simulink model "myFOC"  (R2024b)
settings: Solver=VariableStepAuto  StartTime=0.0  StopTime=6  RelTol=1e-3
InitFcn:
  | init_param;
undefined symbols (not defined in the file): DiscIntNeverNeededParam, inverter, Ki_id, Ki_iq, Kp_id, Kp_iq, PI_params, pmsm, Ts, Ts_motor, Ts_simulink
libraries: mcbcontrolslib x8, simulink x3, slpidlib x1, mcbpmsmnonlinearlib x1, autolibpmsminterior x1
settings Model: Creator=RUSHI JARIWALA  LastModifiedBy=admin
settings SolverCC: AlgebraicLoopSolver=TrustRegion
settings DebuggingCC: UnconnectedInputMsg=warning  UnconnectedOutputMsg=warning  UnconnectedLineMsg=warning
settings ModelReferenceCC: EnableRefExpFcnMdlSchedulingChecks=on
settings RTWCC: GPUComputeCapability=3.5

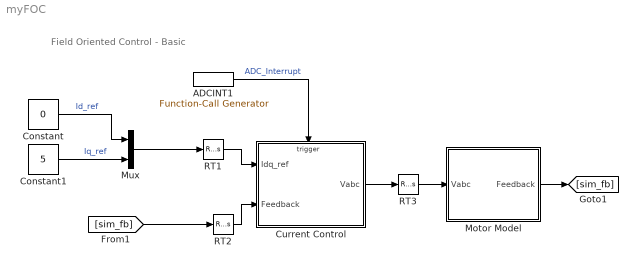
== system myFOC ==
  note: Field Oriented Control - Basic
  ADCINT1 : simulink/Ports & Subsystems/Function-Call Generator  sample_time=Ts  numberOfIterations=1  DisallowWideOutput=off
  Constant : Constant  Value=0  OutDataTypeStr=single
  Constant1 : Constant  Value=5  OutDataTypeStr=single
  Current Control : Subsystem
      settings: RTWSystemCode=Nonreusable function
  Motor Model : Subsystem
  Mux : Mux  Inputs=2
  RT1 : RateTransition  Deterministic=off
  RT2 : RateTransition  Deterministic=off
  RT3 : RateTransition  Deterministic=off
  wires:
  RT2/1 -> Current Control/2(Feedback)
  RT1/1 -> Current Control/1(Idq_ref)
  [sim_fb] -> RT2/1
  Mux/1 -> RT1/1
  Constant/1 -> Mux/1  "Id_ref"
  RT3/1 -> Motor Model/1(Vabc)
  Motor Model/1(Feedback) -> [sim_fb]
  Current Control/1(Vabc) -> RT3/1
  Constant1/1 -> Mux/2  "Iq_ref"
  ADCINT1/1 -> Current Control/Trigger  "ADC_Interrupt"

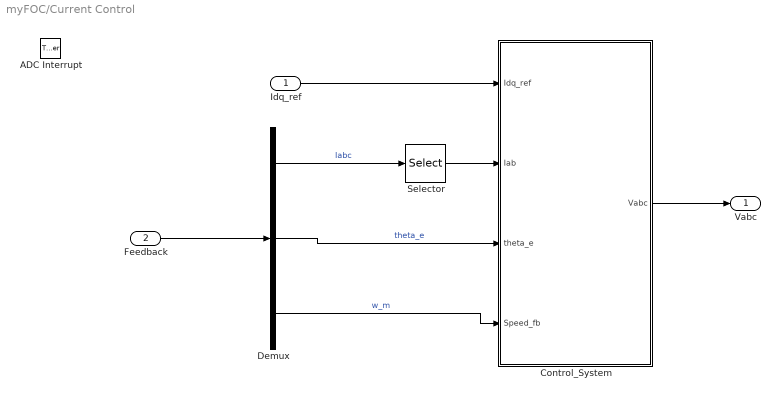
== system myFOC/Current Control ==
  Idq_ref : Inport
  Feedback : Inport  Port=2
  ADC Interrupt : TriggerPort  TriggerType=function-call  VariantControl=Variant
  Control_System : Subsystem
  Demux : Demux  Outputs=3
      settings: DisplayOption=none
  Selector : Selector  InputPortWidth=3  IndexOptions=Index vector (dialog)  Indices=[1 2]  OutputSizes=1
  Vabc : Outport  InitialOutput=0  VectorParamsAs1DForOutWhenUnconnected=off
  wires:
  Idq_ref/1 -> Control_System/1(Idq_ref)
  Control_System/1(Vabc) -> Vabc/1
  Demux/3 -> Control_System/4(Speed_fb)  "w_m"
  Feedback/1 -> Demux/1
  Demux/2 -> Control_System/3(theta_e)  "theta_e"
  Demux/1 -> Selector/1  "Iabc"
  Selector/1 -> Control_System/2(Iab)

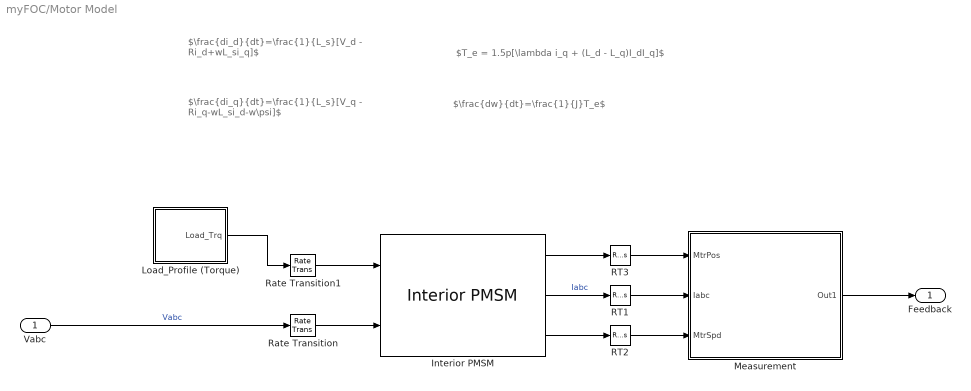
== system myFOC/Motor Model ==
  note: $\frac{dw}{dt}=\frac{1}{J}T_e$
  note: $\frac{di_d}{dt}=\frac{1}{L_s}[V_d - Ri_d+wL_si_q]$
  note: $\frac{di_q}{dt}=\frac{1}{L_s}[V_q - Ri_q-wL_si_d-w\psi]$
  note: $T_e = 1.5p[\lambda i_q + (L_d - L_q)I_dI_q]$
  Vabc : Inport
  Interior PMSM : autolibpmsminterior/Interior PMSM  port_config=Torque  sim_type=Discrete  Ts=Ts_motor  P=pmsm.p  Rs=pmsm.Rs  Ldq=[pmsm.Ld pmsm.Lq]  KConstText=Permanent flux linkage constant (lambda_pm):  lambda_pm=pmsm.FluxPM  Ke=159.9771  mechanical=[pmsm.J, pmsm.B,0]  idq0=[0 0]  theta_init=0  omega_init=0  KConst=pmsm.FluxPM  lambda_pm_calc=pmsm.FluxPM  Kt=0.07  RefBlkName='autolibpmsminterior/Interior PMSM'  aMode=5
      settings: LibrarySourceBlock=mcblib/Electrical Systems/Motors/Interior PMSM
  Load_Profile (Torque) : Subsystem
  Measurement : Subsystem
  RT1 : RateTransition  Deterministic=off  OutPortSampleTime=Ts_simulink
  RT2 : RateTransition  Deterministic=off  OutPortSampleTime=Ts_simulink
  RT3 : RateTransition  Deterministic=off  OutPortSampleTime=Ts_simulink
  Rate Transition : RateTransition  Deterministic=off  OutPortSampleTime=Ts_motor
  Rate Transition1 : RateTransition  Deterministic=off  OutPortSampleTime=Ts_motor
  Feedback : Outport  VectorParamsAs1DForOutWhenUnconnected=off
  wires:
  Measurement/1(Out1) -> Feedback/1
  Interior PMSM/3 -> RT2/1
  RT2/1 -> Measurement/3(MtrSpd)
  RT1/1 -> Measurement/2(Iabc)
  RT3/1 -> Measurement/1(MtrPos)
  Interior PMSM/1 -> RT3/1
  Rate Transition/1 -> Interior PMSM/2
  Vabc/1 -> Rate Transition/1  "Vabc"
  Interior PMSM/2 -> RT1/1  "Iabc"
  Rate Transition1/1 -> Interior PMSM/1
  Load_Profile (Torque)/1(Load_Trq) -> Rate Transition1/1

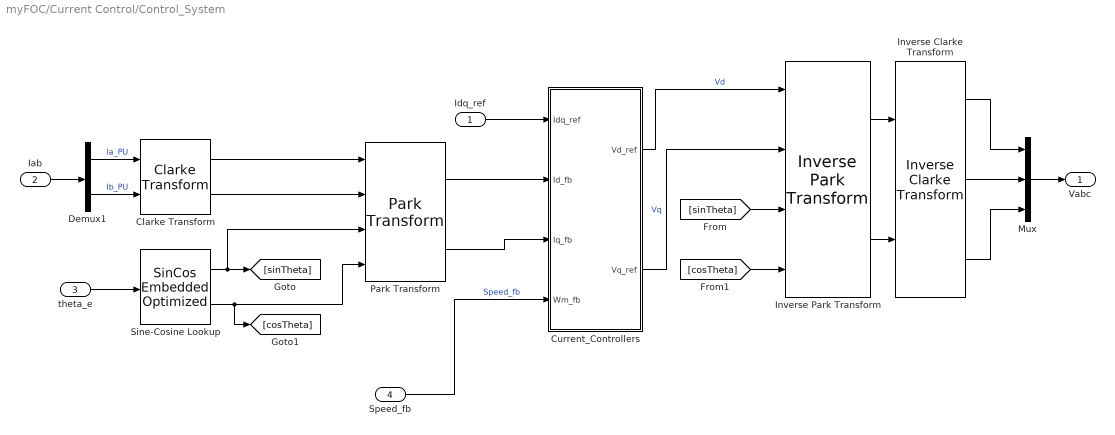
== system myFOC/Current Control/Control_System ==
  Idq_ref : Inport
  Iab : Inport  Port=2
  theta_e : Inport  Port=3
  Speed_fb : Inport  Port=4
  Clarke Transform : mcbcontrolslib/Clarke Transform  VariantControl=Variant2  PhaseInput=Two inputs  EnPowerInv=off
  Current_Controllers : Subsystem
  Demux1 : Demux  Outputs=2
  Inverse Clarke Transform : mcbcontrolslib/Inverse Clarke Transform  PhaseInput=Two inputs  EnPowerInv=off
  Inverse Park Transform : mcbcontrolslib/Inverse Park Transform  PhaseInput=Two inputs  AxisAlignment=D-axis  ThetaInput=Sine and Cosine electrical position  AngleInput=Per-unit  N_points=1024
  Mux : Mux  Inputs=3
  Park Transform : mcbcontrolslib/Park Transform  PhaseInput=Two inputs  AxisAlignment=D-axis  ThetaInput=Sine and Cosine electrical position  AngleInput=Per-unit  N_points=1024
  Sine-Cosine Lookup : mcbcontrolslib/SinCos Embedded Optimized  LabelModeActiveChoice=MCB_Sin  OptforProc=off  ApproximationMethod=None  UserApproxMethod=Lookup  ApproxStatus=None  InterpMethod=Linear point-slope  NumberOfDataPoints=16  NumberOfIterations=11  RemoveProtectionAgainstOutOfRangeInput=off  TableDataTypeStr=Inherit: Inherit via input  AngleInput=Per-unit  ThetaDataType=single  N_points=1024  DatatypeInput=Inherit from input  Datatype=Inherit: Same as input
  Vabc : Outport
  wires:
  Park Transform/1 -> Current_Controllers/2(Id_fb)
  Park Transform/2 -> Current_Controllers/3(Iq_fb)
  Sine-Cosine Lookup/1 -> [sinTheta], Park Transform/3
  Sine-Cosine Lookup/2 -> Park Transform/4, [cosTheta]
  [cosTheta] -> Inverse Park Transform/4
  [sinTheta] -> Inverse Park Transform/3
  Clarke Transform/2 -> Park Transform/2
  Clarke Transform/1 -> Park Transform/1
  Idq_ref/1 -> Current_Controllers/1(Idq_ref)
  Current_Controllers/1(Vd_ref) -> Inverse Park Transform/1  "Vd"
  Current_Controllers/2(Vq_ref) -> Inverse Park Transform/2  "Vq"
  Demux1/1 -> Clarke Transform/1  "Ia_PU"
  Demux1/2 -> Clarke Transform/2  "Ib_PU"
  Iab/1 -> Demux1/1
  Speed_fb/1 -> Current_Controllers/4(Wm_fb)  "Speed_fb"
  theta_e/1 -> Sine-Cosine Lookup/1
  Inverse Park Transform/1 -> Inverse Clarke Transform/1
  Inverse Park Transform/2 -> Inverse Clarke Transform/2
  Inverse Clarke Transform/1 -> Mux/1
  Inverse Clarke Transform/2 -> Mux/2
  Inverse Clarke Transform/3 -> Mux/3
  Mux/1 -> Vabc/1

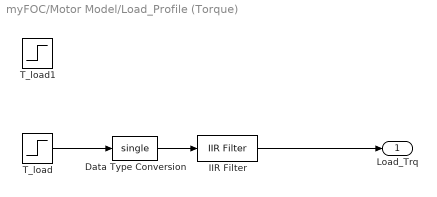
== system myFOC/Motor Model/Load_Profile (Torque) ==
  Data Type Conversion : DataTypeConversion  OutDataTypeStr=single  SaturateOnIntegerOverflow=off  RndMeth=Floor
  IIR Filter : mcbcontrolslib/IIR Filter  VariantControl=Low Pass Filter  VariantSelect=Low-pass  FilterConstantInputType=Specify via dialog  Filter_constant=0.01  advancedSettings=off  Ts=50e-6  cutOff_freq=32.1525
  T_load : Step  Time=5.5  Before=0*pmsm.T_rated  After=0*pmsm.T_rated  SampleTime=Ts_simulink
  T_load1 : Step  Time=2  Before=0.05*pmsm.T_rated  After=-0.05*pmsm.T_rated  SampleTime=Ts_simulink
  Load_Trq : Outport  VectorParamsAs1DForOutWhenUnconnected=off
  wires:
  T_load/1 -> Data Type Conversion/1
  Data Type Conversion/1 -> IIR Filter/1
  IIR Filter/1 -> Load_Trq/1

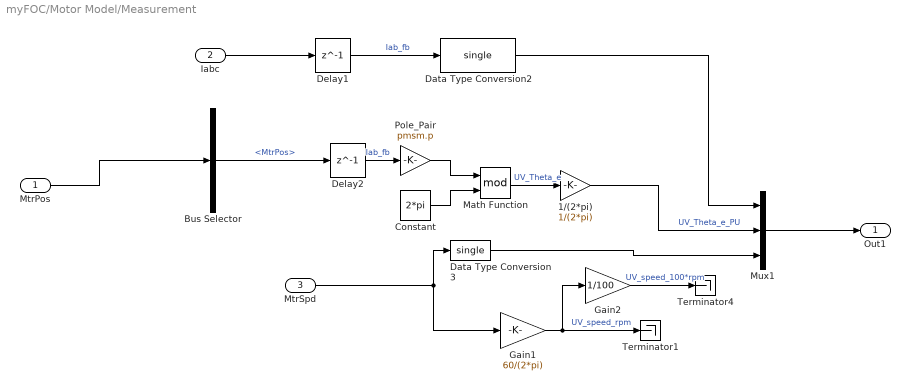
== system myFOC/Motor Model/Measurement ==
  MtrPos : Inport
  Iabc : Inport  Port=2
  MtrSpd : Inport  Port=3
  1/(2*pi) : Gain  Gain=1/(2*pi)  OutDataTypeStr=dataType
  Bus Selector : BusSelector  OutputSignals=MtrPos
  Constant : Constant  Value=2*pi  SampleTime=-1
  Data Type Conversion2 : DataTypeConversion  OutDataTypeStr=single  SaturateOnIntegerOverflow=off  RndMeth=Floor
  Data Type Conversion3 : DataTypeConversion  OutDataTypeStr=single  SaturateOnIntegerOverflow=off  RndMeth=Floor
  Delay1 : Delay  DelayLength=1
  Delay2 : Delay  DelayLength=1
  Gain1 : Gain  Gain=60/(2*pi)  OutDataTypeStr=dataType
  Gain2 : Gain  Gain=1/100  OutDataTypeStr=dataType
  Math Function : Math  Operator=mod
  Mux1 : Mux  Inputs=3
  Pole_Pair : Gain  Gain=pmsm.p
  Terminator1 : Terminator
  Terminator4 : Terminator
  Out1 : Outport
  wires:
  Delay1/1 -> Data Type Conversion2/1  "Iab_fb"
  Delay2/1 -> Pole_Pair/1  "Iab_fb"
  Bus Selector/1 -> Delay2/1  "<MtrPos>"
  Pole_Pair/1 -> Math Function/1
  Constant/1 -> Math Function/2
  Math Function/1 -> 1/(2*pi)/1  "UV_Theta_e"
  1/(2*pi)/1 -> Mux1/2  "UV_Theta_e_PU"
  Mux1/1 -> Out1/1
  MtrSpd/1 -> Gain1/1, Data Type Conversion3/1
  Iabc/1 -> Delay1/1
  MtrPos/1 -> Bus Selector/1
  Gain1/1 -> Gain2/1, Terminator1/1  "UV_speed_rpm"
  Data Type Conversion3/1 -> Mux1/3
  Data Type Conversion2/1 -> Mux1/1
  Gain2/1 -> Terminator4/1  "UV_speed_100*rpm"

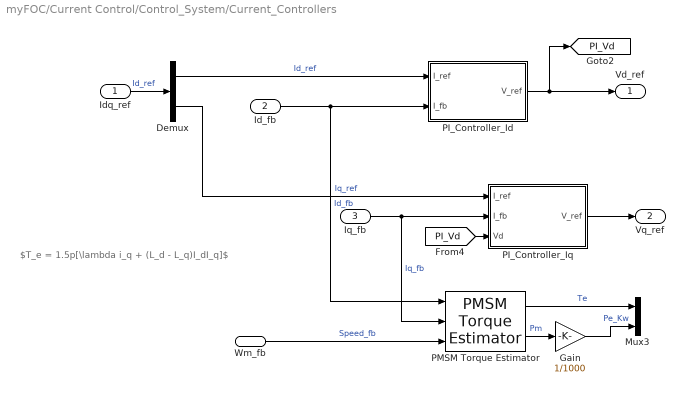
== system myFOC/Current Control/Control_System/Current_Controllers ==
  note: $T_e = 1.5p[\lambda i_q + (L_d - L_q)I_dI_q]$
  Idq_ref : Inport
  Id_fb : Inport  Port=2
  Iq_fb : Inport  Port=3
  Wm_fb : Inport  Port=4
  Demux : Demux  Outputs=2
  Gain : Gain  Gain=1/1000
  Mux3 : Mux  Inputs=2
  PI_Controller_Id : Subsystem
  PI_Controller_Iq : Subsystem
  PMSM Torque Estimator : mcbpmsmnonlinearlib/PMSM Torque Estimator  polePairs=pmsm.p  nonLinearityChoice=Linear model with lumped parameters  Ld=pmsm.Ld  Lq=pmsm.Lq  FluxPM=pmsm.FluxPM  idVec=[-40, -20, 0, 20]  iqVec=[-40, -20, 0, 20, 40]  LdTable=0.2e-3 * ones(4, 5)  LqTable=0.2e-3 * ones(4, 5)  FluxPMTable=6.4e-3 * ones(4, 5)  FluxDTable=[-1.6,-1.6,-1.6,-1.6,-1.6;2.4,2.4,2.4,2.4,2.4;6.4,6.4,6.4,6.4,6.4;10.4,10.4,10.4,10.4,10.4]*1e-3  FluxQTable=[-8,-4,0,4,8;-8,-4,0,4,8;-8,-4,0,4,8;-8,-4,0,4,8]*1e-3  Units=SI Units  V_base=PU_System.V_base  I_base=PU_System.I_base  N_base=PU_System.N_base  T_base=1  P_base=1  scaledTables=on
  Vd_ref : Outport  VectorParamsAs1DForOutWhenUnconnected=off
  Vq_ref : Outport  Port=2  VectorParamsAs1DForOutWhenUnconnected=off
  tag scope: PI_Vd=global
  wires:
  Id_fb/1 -> PMSM Torque Estimator/1, PI_Controller_Id/2(I_fb)  "Id_fb"
  PI_Controller_Iq/1(V_ref) -> Vq_ref/1
  PMSM Torque Estimator/1 -> Mux3/1  "Te"
  Iq_fb/1 -> PMSM Torque Estimator/2, PI_Controller_Iq/2(I_fb)  "Iq_fb"
  Idq_ref/1 -> Demux/1  "Id_ref"
  Wm_fb/1 -> PMSM Torque Estimator/3  "Speed_fb"
  Demux/1 -> PI_Controller_Id/1(I_ref)  "Id_ref"
  Demux/2 -> PI_Controller_Iq/1(I_ref)  "Iq_ref"
  [PI_Vd] -> PI_Controller_Iq/3(Vd)
  PMSM Torque Estimator/2 -> Gain/1  "Pm"
  Gain/1 -> Mux3/2  "Pe_Kw"
  PI_Controller_Id/1(V_ref) -> Vd_ref/1, [PI_Vd]

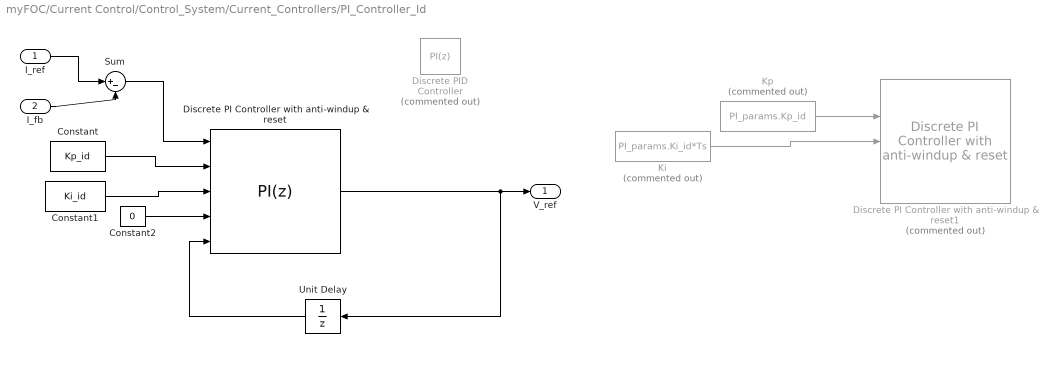
== system myFOC/Current Control/Control_System/Current_Controllers/PI_Controller_Id ==
  I_ref : Inport
  I_fb : Inport  Port=2
  Constant : Constant  Value=Kp_id  OutDataTypeStr=single  SampleTime=-1
  Constant1 : Constant  Value=Ki_id  OutDataTypeStr=single  SampleTime=-1
  Constant2 : Constant  Value=0
  Discrete PI Controller with anti-windup & reset : slpidlib/PID Controller  Controller=PI  Form=Parallel  TimeDomain=Discrete-time  UseExternalTs=off  SampleTime=-1  IntegratorMethod=Forward Euler  FilterMethod=Forward Euler  ControllerParametersSource=external  P=1  I=1  UseKiTs=on  D=0  UseExternalDerivativeSource=off  N=100  UseFilter=on  TunerSelectOption=Transfer Function Based (PID Tuner App)  InitialConditionSource=external  InitialConditionForIntegrator=0  InitialConditionForFilter=0  DifferentiatorICPrevScaledInput=0  ExternalReset=level  TrackingMode=off  Kt=1  LimitOutput=on  SatLimitsSource=internal  UpperSaturationLimit=0.95*inverter.V_dc/sqrt(3)  LowerSaturationLimit=-0.95*inverter.V_dc/sqrt(3)  LinearizeAsGain=on  AntiWindupMode=clamping  Kb=1  LimitIntegrator=off  UpperIntegratorSaturationLimit=inf  LowerIntegratorSaturationLimit=-inf  RndMeth=Simplest  POutMin=[]  POutMax=[]  IOutMin=[]  IOutMax=[]  DOutMin=[]  DOutMax=[]  NOutMin=[]  NOutMax=[]  SumOutMin=[]  SumOutMax=[]  SaturationOutDataTypeStr=Inherit: Inherit via back propagation  SaturationOutMin=[]  SaturationOutMax=[]  PParamMin=[]  PParamMax=[]  IParamMin=[]  IParamMax=[]  DParamMin=[]  DParamMax=[]  NParamMin=[]  NParamMax=[]  KbParamMin=[]  KbParamMax=[]  KtParamMin=[]  KtParamMax=[]  KbOutMin=[]  KbOutMax=[]  KtOutMin=[]  KtOutMax=[]  IntegratorOutMin=[]  IntegratorOutMax=[]  FilterOutMin=[]  FilterOutMax=[]  SumI1OutMin=[]  SumI1OutMax=[]  SumI2OutMin=[]  SumI2OutMax=[]  SumI3OutMin=[]  SumI3OutMax=[]  SumI4OutMin=[]  SumI4OutMax=[]  SumDOutMin=[]  SumDOutMax=[]  DifferentiatorOutMin=[]  DifferentiatorOutMax=[]  FilterDiffOutCoefMin=[]  FilterDiffOutCoefMax=[]  ReciprocalOutMin=[]  ReciprocalOutMax=[]  SumDenOutMin=[]  SumDenOutMax=[]  SumNumOutMin=[]  SumNumOutMax=[]  DivideOutMin=[]  DivideOutMax=[]  UdiffTsProdOutMin=[]  UdiffTsProdOutMax=[]  NTsProdOutMin=[]  NTsProdOutMax=[]  UintegralTsProdOutMin=[]  UintegralTsProdOutMax=[]  UngainTsProdOutMin=[]  UngainTsProdOutMax=[]  ClampingZeroOutDataTypeStr=Inherit: Inherit via back propagation  ClampingZeroOutMin=[]  ClampingZeroOutMax=[]  FilterDenConstantOutDataTypeStr=Inherit: Inherit via back propagation  FilterDenConstantOutMin=[]  FilterDenConstantOutMax=[]  PCopyOutDataTypeStr=Inherit: Inherit via back propagation  PCopyOutMin=[]  PCopyOutMax=[]  NCopyOutDataTypeStr=Inherit: Inherit via back propagation  NCopyOutMin=[]  NCopyOutMax=[]  IntegratorContinuousStateAttributes=''  IntegratorStateMustResolveToSignalObject=off  IntegratorRTWStateStorageClass=Auto  FilterContinuousStateAttributes=''  FilterStateMustResolveToSignalObject=off  FilterRTWStateStorageClass=Auto  ParallelPVariant=ExternalParameters  IdealPVariant=Disabled  IVariant=ExternalParameters  DVariant=Disabled  IntegratorVariant=Discrete  SatVariant=Enabled  AWVariant=DiscClampingParallel  PCopyVariant=Disabled  TRVariant=Disabled  FdbkBlocksVariant=Forward  IdealPFdbkVariant=Disabled  SatFdbkVariant=Disabled  DerivativeFilterVariant=Disabled  NVariant=Disabled  NCopyVariant=Disabled_SignalSpec  FilterICVariant=Disabled  IntegratorICVariant=ExternalICs  ExternalResetVariant=ExternalReset  TRSumVariant=Passthrough  SumFdbkVariant=Disabled  SumVariant=Sum_PI  TsampFilterVariant=InternalTs  TsampNgainVariant=Passthrough  TsampIntegralVariant=Disabled_SignalSpec  ExternalSaturationOutDataTypeStr=Inherit: Same as second input  DerivativeSourceVariant=Disabled  PreIntVariant=InternalPreInt
      settings: LibrarySourceBlock=mcbcontrolslib/PI Controller
  Discrete PI Controller with anti-windup & reset1 : mcbcontrolslib/Discrete PI Controller  with anti-windup & reset  Commented=on  UpperSaturationLimit=1  LowerSaturationLimit=-1
  Discrete PID Controller : simulink/Continuous/PID Controller  Commented=on  Controller=PI  Form=Parallel  TimeDomain=Discrete-time  UseExternalTs=off  SampleTime=-1  IntegratorMethod=Forward Euler  FilterMethod=Forward Euler  ControllerParametersSource=internal  P=1  I=1  D=0  UseFilter=on  N=100  TunerSelectOption=Transfer Function Based (PID Tuner App)  InitialConditionSource=internal  InitialConditionForIntegrator=0  InitialConditionForFilter=0  DifferentiatorICPrevScaledInput=0  ExternalReset=none  TrackingMode=off  Kt=1  LimitOutput=off  UpperSaturationLimit=inf  LowerSaturationLimit=-inf  LinearizeAsGain=off  AntiWindupMode=none  Kb=1  POutMin=[]  POutMax=[]  IOutMin=[]  IOutMax=[]  DOutMin=[]  DOutMax=[]  NOutMin=[]  NOutMax=[]  SumOutMin=[]  SumOutMax=[]  SaturationOutMin=[]  SaturationOutMax=[]  PParamMin=[]  PParamMax=[]  IParamMin=[]  IParamMax=[]  DParamMin=[]  DParamMax=[]  NParamMin=[]  NParamMax=[]  KbParamMin=[]  KbParamMax=[]  KtParamMin=[]  KtParamMax=[]  KbOutMin=[]  KbOutMax=[]  KtOutMin=[]  KtOutMax=[]  IntegratorOutMin=[]  IntegratorOutMax=[]  FilterOutMin=[]  FilterOutMax=[]  SumI1OutMin=[]  SumI1OutMax=[]  SumI2OutMin=[]  SumI2OutMax=[]  SumI3OutMin=[]  SumI3OutMax=[]  SumI4OutMin=[]  SumI4OutMax=[]  SumDOutMin=[]  SumDOutMax=[]  DifferentiatorOutMin=[]  DifferentiatorOutMax=[]  FilterDiffOutCoefMin=[]  FilterDiffOutCoefMax=[]  ReciprocalOutMin=[]  ReciprocalOutMax=[]  SumDenOutMin=[]  SumDenOutMax=[]  SumNumOutMin=[]  SumNumOutMax=[]  DivideOutMin=[]  DivideOutMax=[]  UdiffTsProdOutMin=[]  UdiffTsProdOutMax=[]  NTsProdOutMin=[]  NTsProdOutMax=[]  UintegralTsProdOutMin=[]  UintegralTsProdOutMax=[]  UngainTsProdOutMin=[]  UngainTsProdOutMax=[]  IntegratorContinuousStateAttributes=''  IntegratorStateMustResolveToSignalObject=off  IntegratorRTWStateStorageClass=Auto  FilterContinuousStateAttributes=''  FilterStateMustResolveToSignalObject=off  FilterRTWStateStorageClass=Auto  ParallelPVariant=InternalParameters  IdealPVariant=Disabled  IVariant=InternalParameters  DVariant=Disabled  IntegratorVariant=Discrete  SatVariant=Disabled  AWVariant=Passthrough  PCopyVariant=Disabled  TRVariant=Disabled  FdbkBlocksVariant=Forward  IdealPFdbkVariant=Disabled  SatFdbkVariant=Disabled  DerivativeFilterVariant=Disabled  NVariant=Disabled  NCopyVariant=Disabled_SignalSpec  FilterICVariant=Disabled  IntegratorICVariant=InternalICs  ExternalResetVariant=Disabled  TRSumVariant=Passthrough  SumFdbkVariant=Disabled  SumVariant=Sum_PI  TsampFilterVariant=InternalTs  TsampNgainVariant=Passthrough  TsampIntegralVariant=Passthrough
  Ki : Constant  Commented=on  Value=PI_params.Ki_id*Ts  OutDataTypeStr=dataType  SampleTime=-1
  Kp : Constant  Commented=on  Value=PI_params.Kp_id  OutDataTypeStr=dataType  SampleTime=-1
  Sum : Sum  Inputs=|+-  OutDataTypeStr=Inherit: Same as first input
  Unit Delay : UnitDelay  SampleTime=-1  HasFrameUpgradeWarning=on
  V_ref : Outport  VectorParamsAs1DForOutWhenUnconnected=off
  wires:
  I_fb/1 -> Sum/2
  I_ref/1 -> Sum/1
  Unit Delay/1 -> Discrete PI Controller with anti-windup & reset/5
  Sum/1 -> Discrete PI Controller with anti-windup & reset/1
  Discrete PI Controller with anti-windup & reset/1 -> Unit Delay/1, V_ref/1
  Constant/1 -> Discrete PI Controller with anti-windup & reset/2
  Constant1/1 -> Discrete PI Controller with anti-windup & reset/3
  Kp/1 -> Discrete PI Controller with anti-windup & reset1/2
  Ki/1 -> Discrete PI Controller with anti-windup & reset1/3
  Constant2/1 -> Discrete PI Controller with anti-windup & reset/4

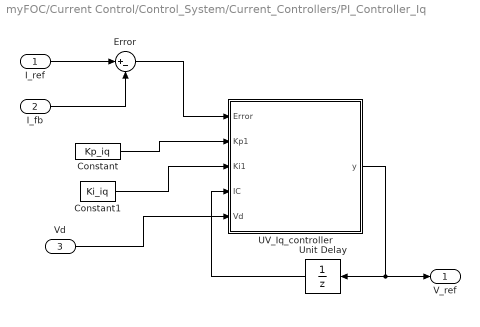
== system myFOC/Current Control/Control_System/Current_Controllers/PI_Controller_Iq ==
  I_ref : Inport
  I_fb : Inport  Port=2
  Vd : Inport  Port=3
  Constant : Constant  Value=Kp_iq  OutDataTypeStr=single  SampleTime=-1
  Constant1 : Constant  Value=Ki_iq  OutDataTypeStr=single  SampleTime=-1
  Error : Sum  Inputs=|+-  OutDataTypeStr=Inherit: Same as first input
  UV_Iq_controller : Subsystem
  Unit Delay : UnitDelay  SampleTime=-1  HasFrameUpgradeWarning=on
  V_ref : Outport  VectorParamsAs1DForOutWhenUnconnected=off
  wires:
  I_fb/1 -> Error/2
  I_ref/1 -> Error/1
  Error/1 -> UV_Iq_controller/1(Error)
  UV_Iq_controller/1(y) -> V_ref/1, Unit Delay/1
  Constant/1 -> UV_Iq_controller/2(Kp1)
  Constant1/1 -> UV_Iq_controller/3(Ki1)
  Vd/1 -> UV_Iq_controller/5(Vd)
  Unit Delay/1 -> UV_Iq_controller/4(IC)

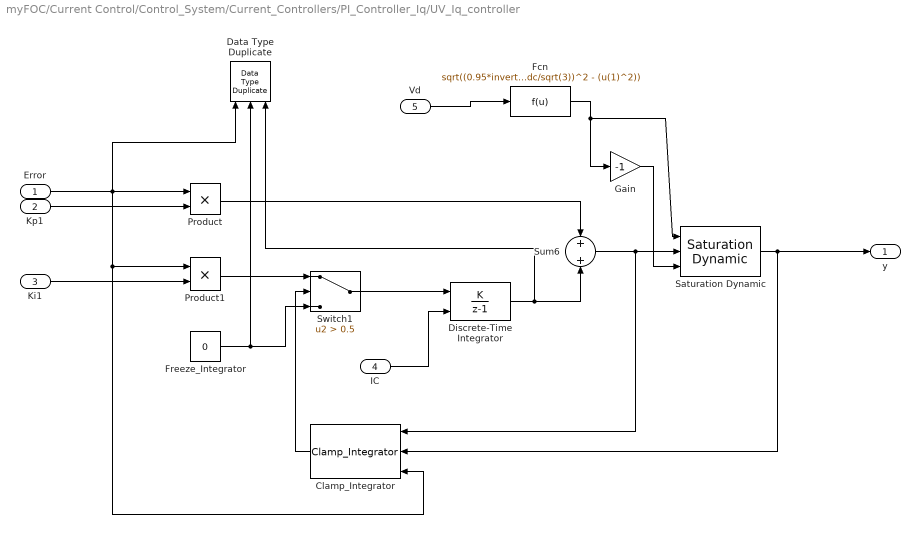
== system myFOC/Current Control/Control_System/Current_Controllers/PI_Controller_Iq/UV_Iq_controller ==
  Error : Inport
  Kp1 : Inport  Port=2
  Ki1 : Inport  Port=3
  IC : Inport  Port=4
  Vd : Inport  Port=5
  Clamp_Integrator : mcbcontrolslib/Discrete PI Controller  with anti-windup & reset/Clamp_Integrator  SystemSampleTime=-1  Latency=0  AutoFrameSizeCalculation=off
  Data Type Duplicate : DataTypeDuplicate  NumInputPorts=3
  Discrete-Time Integrator : DiscreteIntegrator  IntegratorMethod=Accumulation: Forward Euler  InitialConditionSource=external  SampleTime=-1  OutDataTypeStr=Inherit: Inherit via back propagation  RndMeth=Simplest  ICPrevOutput=DiscIntNeverNeededParam  ICPrevScaledInput=DiscIntNeverNeededParam
  Fcn : Fcn  Expr=sqrt((0.95*inverter.V_dc/sqrt(3))^2 - (u(1)^2))
  Freeze_Integrator : Constant  Value=0  OutDataTypeStr=Inherit: Inherit via back propagation  SampleTime=-1
  Gain : Gain  Gain=-1  OutDataTypeStr=single
  Product : Product  RndMeth=Simplest  OutDataTypeStr=Inherit: Same as first input
  Product1 : Product  RndMeth=Simplest  OutDataTypeStr=Inherit: Same as first input
  Saturation Dynamic : simulink/Discontinuities/Saturation Dynamic  OutMin=[]  OutMax=[]  OutDataTypeStr=Inherit: Same as second input  OutDataType=fixdt(1, 16)  OutScaling=2^-10  DoSatur=off
  Sum6 : Sum  InputSameDT=on  RndMeth=Simplest  OutDataTypeStr=Inherit: Same as first input
  Switch1 : Switch  Criteria=u2 > Threshold  Threshold=0.5  OutDataTypeStr=Inherit: Inherit via back propagation  RndMeth=Simplest  ZeroCross=off  SaturateOnIntegerOverflow=off  InputSameDT=off
  y : Outport
  wires:
  Clamp_Integrator/1 -> Switch1/2
  Freeze_Integrator/1 -> Switch1/3, Data Type Duplicate/2
  Fcn/1 -> Saturation Dynamic/1, Gain/1
  Error/1 -> Data Type Duplicate/1, Product/1, Product1/1, Clamp_Integrator/3
  Vd/1 -> Fcn/1
  Saturation Dynamic/1 -> y/1, Clamp_Integrator/2
  Ki1/1 -> Product1/2
  Discrete-Time Integrator/1 -> Sum6/2, Data Type Duplicate/3
  Product/1 -> Sum6/1
  Kp1/1 -> Product/2
  Sum6/1 -> Saturation Dynamic/2, Clamp_Integrator/1
  Product1/1 -> Switch1/1
  IC/1 -> Discrete-Time Integrator/2
  Switch1/1 -> Discrete-Time Integrator/1
  Gain/1 -> Saturation Dynamic/3
